simulink model "Spring_mass_damper_system"  (R2023b)
settings: Solver=VariableStepAuto  StartTime=0.0  StopTime=10  MaxStep=0.01  RelTol=1e-3
settings Model: Creator=91839  LastModifiedBy=siva kumar
settings SolverCC: AlgebraicLoopSolver=TrustRegion
settings DataIOCC: ExternalInput=data  SaveFormat=Array  DSMLogging=off  ReturnWorkspaceOutputs=off
settings DebuggingCC: UnconnectedInputMsg=warning  UnconnectedOutputMsg=warning  UnconnectedLineMsg=warning
settings ModelReferenceCC: EnableRefExpFcnMdlSchedulingChecks=on
settings SFSimCC: CustomCodeUndefinedFunction=UseInterfaceOnly

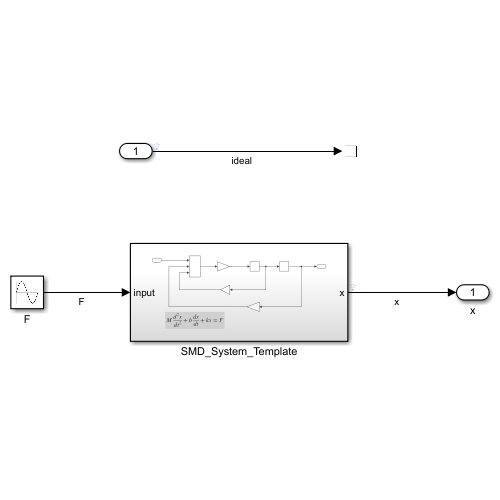
[thumbnail: Simulink's stored preview of the top-level diagram]
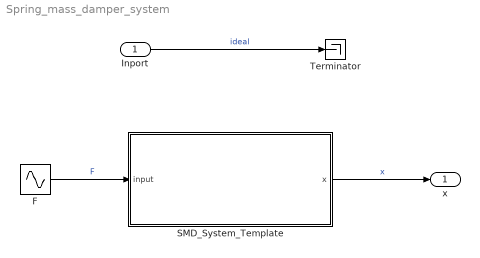
== system Spring_mass_damper_system ==
  Inport : Inport
  F : Sin  SampleTime=0
  SMD_System_Template : Subsystem
  Terminator : Terminator
  x : Outport
  wires:
  Inport/1 -> Terminator/1  "ideal"
  F/1 -> SMD_System_Template/1(input)  "F"
  SMD_System_Template/1(x) -> x/1  "x"

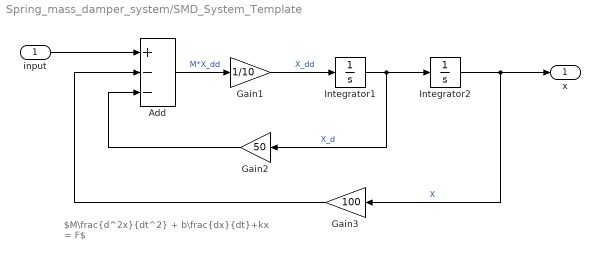
== system Spring_mass_damper_system/SMD_System_Template ==
  note: $M\frac{d^2x}{dt^2} + b\frac{dx}{dt}+kx = F$
  input : Inport
  Add : Sum  Inputs=+--
  Gain1 : Gain  Gain=1/10
  Gain2 : Gain  Gain=50
  Gain3 : Gain  Gain=100
  Integrator1 : Integrator
  Integrator2 : Integrator
  x : Outport
  wires:
  Add/1 -> Gain1/1  "M*X_dd"
  Gain1/1 -> Integrator1/1  "X_dd"
  Integrator1/1 -> Integrator2/1, Gain2/1  "X_d"
  Integrator2/1 -> x/1, Gain3/1  "X"
  Gain2/1 -> Add/3
  Gain3/1 -> Add/2
  input/1 -> Add/1
